simulink model "SourcesTest"  (R2021a)
settings: Solver=FixedStepDiscrete  StartTime=0.0  StopTime=inf  RelTol=1e-3
libraries: simulink x3
settings Model: Creator=Michael_Ibrahim  LastModifiedBy=Michael_Ibrahim
settings OptimizationCC: DefaultParameterBehavior=Inlined  InlineInvariantSignals=on  EnhancedBackFolding=on  PassReuseOutputArgsAs=Individual arguments  ZeroExternalMemoryAtStartup=off  ZeroInternalMemoryAtStartup=off  OptimizeBlockOrder=speed  DifferentSizesBufferReuse=on  OptimizationCustomize=off  EfficientTunableParamExpr=on
settings DebuggingCC: UnderspecifiedInitializationDetection=Classic  MergeDetectMultiDrivingBlocksExec=none  ParameterTunabilityLossMsg=error
settings ModelReferenceCC: PropagateSignalLabelsOutOfModel=off
settings SFSimCC: MATLABDynamicMemAlloc=off
settings RTWCC: SystemTargetFile=ert.tlc  GenCodeOnly=on  TemplateMakefile=ert_default_tmf  GenerateReport=on  IncludeHyperlinkInReport=on  LaunchReport=on  GenerateTraceInfo=on  GenerateTraceReport=on  GenerateTraceReportSl=on  GenerateTraceReportSf=on  GenerateTraceReportEml=on
settings CodeAppCC: ForceParamTrailComments=on  IgnoreCustomStorageClasses=off  OperatorAnnotations=on  SimulinkDataObjDesc=on  SFDataObjDesc=on  InsertBlockDesc=on
settings ERTTargetCC: TargetLangStandard=C99 (ISO)  GenerateSampleERTMain=on  InlinedParameterPlacement=NonHierarchical  ERTCustomFileTemplate=example_file_process.tlc

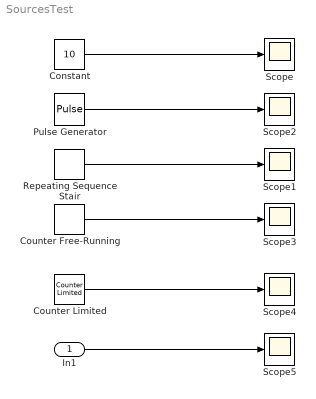
== system SourcesTest ==
  In1 : Inport
  Constant : Constant  Value=10  OutDataTypeStr=uint8  SampleTime=1  LockScale=on
  Counter Free-Running : simulink/Sources/Counter Free-Running  NumBits=3  tsamp=1
  Counter Limited : simulink/Sources/Counter Limited  uplimit=5  tsamp=1
  Pulse Generator : DiscretePulseGenerator  Period=10  PulseWidth=5  SampleTime=0.5
  Repeating Sequence Stair : simulink/Sources/Repeating Sequence Stair  OutValues=[1 3 5 7 3]  tsamp=1  OutMin=[]  OutMax=[]  OutDataTypeStr=double  OutputDataTypeScalingMode=double  OutDataType=fixdt(0,8)  ConRadixGroup=Best Precision: Vector-wise  OutScaling=2^-12
  Scope{,1..5} (6 alike) : Scope
  wires:
  Constant/1 -> Scope/1
  Pulse Generator/1 -> Scope2/1
  Repeating Sequence Stair/1 -> Scope1/1
  Counter Free-Running/1 -> Scope3/1
  Counter Limited/1 -> Scope4/1
  In1/1 -> Scope5/1
